simulink model "Session2_PID_OS_simulink"  (R2014a)
settings: Solver=ode45  StartTime=0.0  StopTime=10.0  RelTol=1e-3
values from neighbouring files (symbols this model uses):
  wn = 2    [Session2_PID_OS.m]
  Zeta = 0.3    [Session2_PID_OS.m]
settings Model: Creator=Omar Emad  LastModifiedBy=Omar Emad

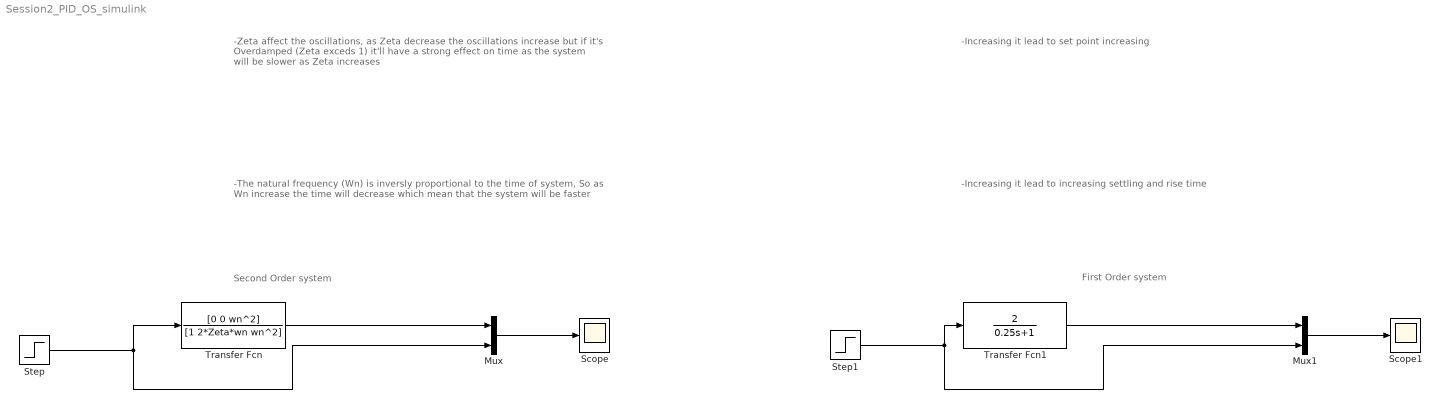
== system Session2_PID_OS_simulink ==
  note: -Zeta affect the oscillations, as Zeta decrease the oscillations increase
      | but if it's Overdamped (Zeta exceds 1) it'll have a strong effect on time
      | as the system will be slower as Zeta increases
  note: First Order system
  note: Second Order system
  note: -The natural frequency (Wn) is inversly proportional to the time of
      | system, So as Wn increase the time will decrease which mean that the
      | system will be faster
  note: -Increasing it lead to set point increasing
  note: -Increasing it lead to increasing settling and rise time
  Mux : Mux  Inputs=2
  Mux1 : Mux  Inputs=2
  Scope : Scope
  Scope1 : Scope
  Step : Step  SampleTime=0
  Step1 : Step  SampleTime=0
  Transfer Fcn : TransferFcn  Numerator=[0 0 wn^2]  Denominator=[1 2*Zeta*wn wn^2]
  Transfer Fcn1 : TransferFcn  Numerator=[2]  Denominator=[0.25 1]
  wires:
  Step/1 -> Transfer Fcn/1, Mux/2
  Transfer Fcn/1 -> Mux/1
  Mux/1 -> Scope/1
  Step1/1 -> Transfer Fcn1/1, Mux1/2
  Transfer Fcn1/1 -> Mux1/1
  Mux1/1 -> Scope1/1
